simulink model "PENDULUM"  (R2017a)
settings: Solver=VariableStepAuto  StartTime=0.0  StopTime=20.0  RelTol=1e-3
libraries: dspsrcs4 x1
settings Model: Creator=Marco  LastModifiedBy=Marco

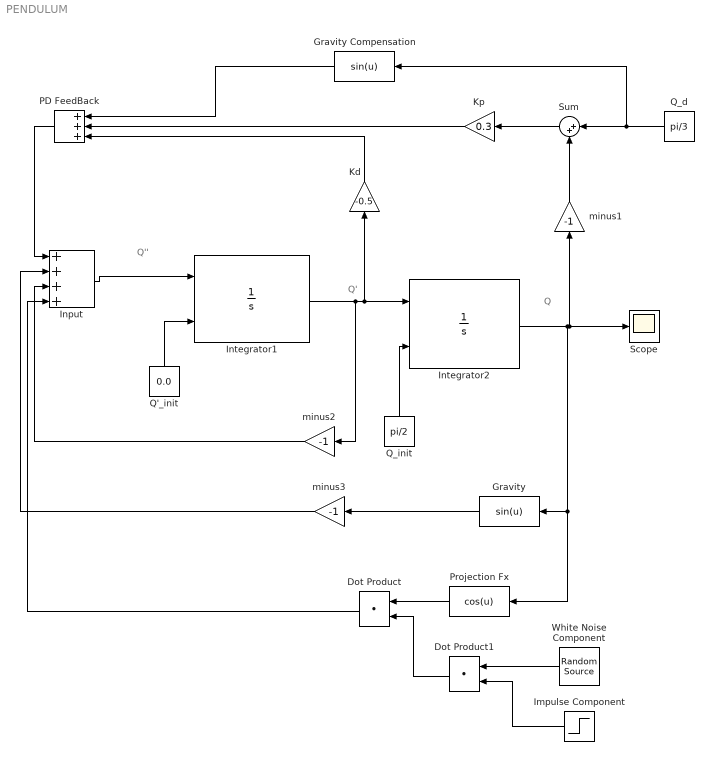
== system PENDULUM ==
  note: Q
  note: Q'
  note: Q''
  Dot Product : DotProduct  InputSameDT=on  OutDataTypeStr=Inherit: Inherit via internal rule
  Dot Product1 : DotProduct  InputSameDT=on  OutDataTypeStr=Inherit: Inherit via internal rule
  "Gravity " : Fcn  Expr=sin(u)
  Gravity Compensation : Fcn  Expr=sin(u)
  Impulse Component : Step  Time=5  Before=5  After=0  SampleTime=0
  Input : Sum  Inputs=++++
  Integrator1 : Integrator  InitialConditionSource=external
  "Integrator2 " : Integrator  InitialConditionSource=external
  Kd : Gain  Gain=-0.5
  Kp : Gain  Gain=0.3
  PD FeedBack : Sum  Inputs=+++
  Projection Fx : Fcn  Expr=cos(u)
  Q'_init : Constant  Value=0.0
  Q_d : Constant  Value=pi/3
  Q_init : Constant  Value=pi/2
  Scope : Scope
  Sum : Sum  Inputs=|++
  White Noise Component : dspsrcs4/Random Source  SrcType=Gaussian  NormMethod=Ziggurat  CltLength=12  MinVal=0  MaxVal=1  MeanVal=0  VarVal=1  RepMode=Not repeatable  rawSeed=1  IsInherit=off  SampMode=Discrete  SampTime=1  SampFrame=1  DataType=Double  OutComplex=Real  OutputFrames=off
  minus1 : Gain  Gain=-1
  minus2 : Gain  Gain=-1
  minus3 : Gain  Gain=-1
  wires:
  Integrator1/1 -> minus2/1, Kd/1, "Integrator2 "/1
  "Gravity "/1 -> minus3/1
  "Integrator2 "/1 -> Projection Fx/1, "Gravity "/1, minus1/1, Scope/1
  minus3/1 -> Input/2
  minus2/1 -> Input/3
  Input/1 -> Integrator1/1
  Q_init/1 -> "Integrator2 "/2
  Q'_init/1 -> Integrator1/2
  Q_d/1 -> Gravity Compensation/1, Sum/1
  minus1/1 -> Sum/2
  PD FeedBack/1 -> Input/1
  Kd/1 -> PD FeedBack/3
  Sum/1 -> Kp/1
  Kp/1 -> PD FeedBack/2
  Gravity Compensation/1 -> PD FeedBack/1
  Projection Fx/1 -> Dot Product/1
  Dot Product/1 -> Input/4
  White Noise Component/1 -> Dot Product1/1
  Impulse Component/1 -> Dot Product1/2
  Dot Product1/1 -> Dot Product/2
